simulink model "motor_simulation"  (Simulink 10.2)
settings: Solver=FixedStepAuto  StartTime=0.0  StopTime=0.6  FixedStep=0.000001  RelTol=1e-3
values from neighbouring files (symbols this model uses):
  Ki = K/T    (= 19.1865109557)    [set_parameters.m]
  Ki2 = 100    [set_parameters.m]
  Kp = K    (= -0.346424796047)    [set_parameters.m]
  Kp2 = 200.0    (= 200)    [set_parameters.m]
  L = 0.00054    [set_parameters.m]
  R = 0.55    [set_parameters.m]
settings Model: Creator=omicron  LastModifiedBy=omicron
settings DataIOCC: SaveFormat=Dataset  SignalLoggingSaveFormat=Dataset  ReturnWorkspaceOutputs=on
settings OptimizationCC: LifeSpan=auto
settings DebuggingCC: UnderspecifiedInitializationDetection=Simplified  MergeDetectMultiDrivingBlocksExec=error  FcnCallInpInsideContextMsg=error  SFUnexpectedBacktrackingDiag=error  SFNoUnconditionalDefaultTransitionDiag=error  SFExecutionAtInitializationDiag=warning  ArithmeticOperatorsInVariantConditions=error
settings HardwareCC: ProdBitPerPointer=64  ProdBitPerSizeT=64  ProdBitPerPtrDiffT=64  ProdLargestAtomicFloat=Float  ProdIntDivRoundTo=Zero  ProdEndianess=LittleEndian  ProdWordSize=64  ProdHWDeviceType=Intel->x86-64 (Windows64)
settings ModelReferenceCC: PropagateSignalLabelsOutOfModel=on
settings SFSimCC: SimUseLocalCustomCode=on  CustomCodeUndefinedFunction=FilterOut
settings RTWCC: RTWUseLocalCustomCode=on
settings CodeAppCC: StateflowObjectComments=off
settings GRTTargetCC: TargetLangStandard=C99 (ISO)  CombineOutputUpdateFcns=on  GRTInterface=off
settings ConfigComp: CovMetricSettings=dwe  CovSaveCumulativeToWorkspaceVar=off  CovSaveSingleToWorkspaceVar=off  CovExternalEMLEnable=on

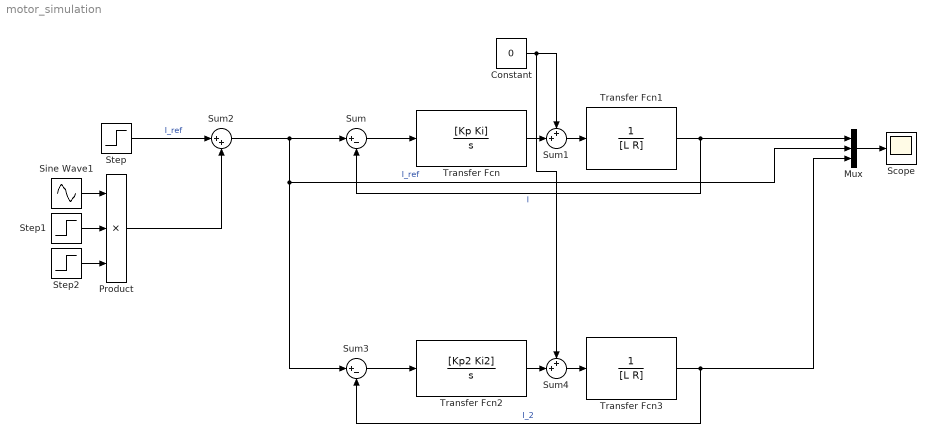
== system motor_simulation ==
  Constant : Constant  Value=0
  Mux : Mux  Inputs=3
  Product : Product  Inputs=3
  Scope : Scope
  Sine Wave1 : Sin  Frequency=50  Phase=-0.15  SampleTime=0
  Step : Step  Time=0.05  SampleTime=0
  Step1 : Step  Time=0.15  SampleTime=0
  Step2 : Step  Time=0.4  Before=1  After=0  SampleTime=0
  Sum : Sum  Inputs=|+-
  Sum1 : Sum  Inputs=++|
  Sum2 : Sum  Inputs=|++
  Sum3 : Sum  Inputs=|+-
  Sum4 : Sum  Inputs=++|
  Transfer Fcn : TransferFcn  Numerator=[Kp Ki]  Denominator=[1 0]
  Transfer Fcn1 : TransferFcn  Denominator=[L R]
  Transfer Fcn2 : TransferFcn  Numerator=[Kp2 Ki2]  Denominator=[1 0]
  Transfer Fcn3 : TransferFcn  Denominator=[L R]
  wires:
  Sum/1 -> Transfer Fcn/1
  Transfer Fcn1/1 -> Mux/1, Sum/2  "I"
  Mux/1 -> Scope/1
  Transfer Fcn/1 -> Sum1/2
  Sum1/1 -> Transfer Fcn1/1
  Sine Wave1/1 -> Product/1
  Step1/1 -> Product/2
  Product/1 -> Sum2/2
  Step/1 -> Sum2/1  "I_ref"
  Constant/1 -> Sum4/1, Sum1/1
  Transfer Fcn2/1 -> Sum4/2
  Sum4/1 -> Transfer Fcn3/1
  Sum2/1 -> Sum3/1, Mux/2, Sum/1  "I_ref"
  Transfer Fcn3/1 -> Mux/3, Sum3/2  "I_2"
  Sum3/1 -> Transfer Fcn2/1
  Step2/1 -> Product/3
